simulink model "Lab3"  (Simulink 7.3)
settings: Solver=ode1  SolverMode=SingleTasking  StartTime=0.0  StopTime=5  FixedStep=0.001  RelTol=1e-3
values from neighbouring files (symbols this model uses):
  Beq = 0.0015*6    (= 0.009)    [Sve ikad.m]    (also in matlab.mat = 0.0075)
  den_k = [1 100*a]    [Sve ikad.m]    (also in matlab.mat = [1 286.356023126])
  Eff_G = 0.9    [Sve ikad.m]    (also in matlab.mat)
  Eff_M = 0.69    [Sve ikad.m]    (also in matlab.mat)
  Jeq = 2e-3    (= 0.002)    [Sve ikad.m]    (also in matlab.mat)
  Ke = 0.0076776    [Sve ikad.m]    (also in matlab.mat)
  Kg = 70    [Sve ikad.m]    (also in matlab.mat)
  Km = 0.007683    [Sve ikad.m]    (also in matlab.mat)
  Kp = 41.5    [Sve ikad.m]    (also in matlab.mat = 160)
  num_k = [1*a 100]    [Sve ikad.m]    (also in matlab.mat = [2.86356023126 100])
  Ra = 2.6    [Sve ikad.m]    (also in matlab.mat)
undefined symbols (not defined in the file or in its folder): MultiQ, PCI, Quanser
libraries: rtwinlib x2
settings Model: Creator=Labos  LastModifiedBy=Mehatronicki Sustavi  SimulationMode=external  ExtModeTrigDuration=1000000
settings HardwareCC: ProdIntDivRoundTo=Zero  ProdEndianess=LittleEndian  ProdHWDeviceType=Generic->32-bit x86 compatible
settings RTWCC: SystemTargetFile=rtwin.tlc  TemplateMakefile=rtwin.tmf  Description=Real-Time Windows Target  ProcessScript=rtwin_make_rtw_hook  RTWCompilerOptimization=On
settings CodeAppCC: MaxIdLength=95
settings RTWinTargetCC: TargetFunctionLibrary=ANSI_C  PortableWordSizes=off

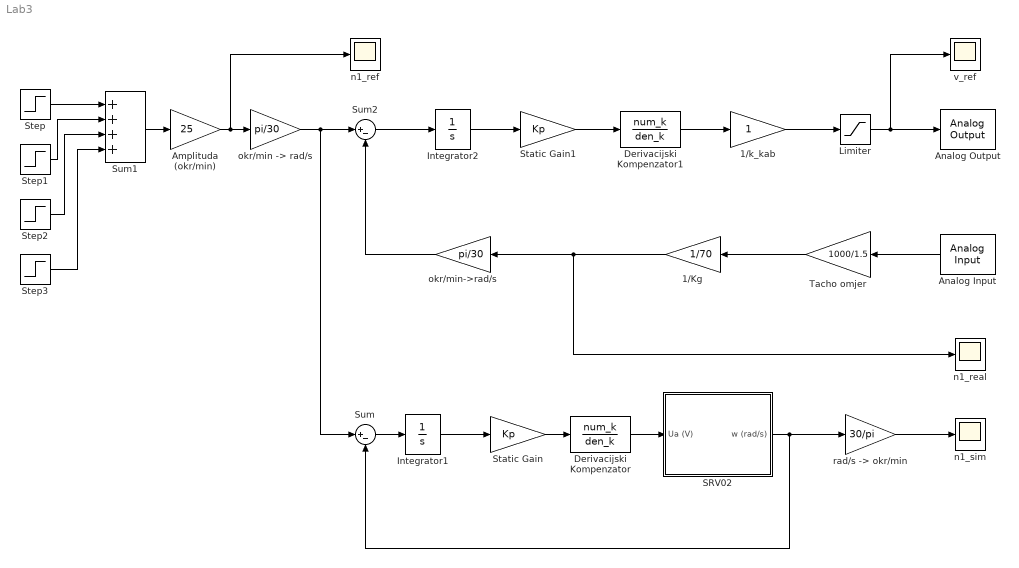
== system Lab3 ==
  1/Kg : Gain  Gain=1/70
  1/k_kab : Gain
  Amplituda (okr/min) : Gain  Gain=25
  Analog Input : rtwinlib/Analog Input  SampleTime=0.001  DrvName=Quanser/MultiQ-PCI  DrvAddress=4294967295  DrvOptions=zeros(1,0)  Channels=4  RangeMode=1  VoltRange=1  DataType=1
      settings: AttributesFormatString=Quanser\nMultiQ-PCI [auto]
  Analog Output : rtwinlib/Analog Output  SampleTime=0.001  DrvName=Quanser/MultiQ-PCI  DrvAddress=4294967295  DrvOptions=zeros(1,0)  Channels=1  RangeMode=1  VoltRange=1  InitialValue=0  FinalValue=0
      settings: AttributesFormatString=Quanser\nMultiQ-PCI [auto]
  Derivacijski Kompenzator : TransferFcn  Numerator=num_k  Denominator=den_k
  Derivacijski Kompenzator1 : TransferFcn  Numerator=num_k  Denominator=den_k
  Integrator1 : Integrator
  Integrator2 : Integrator
  Limiter : Saturate  UpperLimit=6  LowerLimit=-6
  "SRV02 " : Subsystem
  Static Gain : Gain  Gain=Kp
  Static Gain1 : Gain  Gain=Kp
  Step : Step
  Step1 : Step  Time=2  After=-1
  Step2 : Step  Time=3  After=-1
  Step3 : Step  Time=4
  Sum : Sum  Inputs=|+-
  Sum1 : Sum  Inputs=++++
  Sum2 : Sum  Inputs=|+-
  Tacho omjer : Gain  Gain=1000/1.5
  n1_real : Scope
      settings: TimeRange=5  YMin=0  YMax=30  SaveName=n2_real  DataFormat=Array  SampleInput=on
  n1_ref : Scope
      settings: TimeRange=5  YMin=0  YMax=30  SaveName=n2_ref  DataFormat=Array  SampleInput=on
  n1_sim : Scope
      settings: TimeRange=5  YMin=0  YMax=30  SaveName=n2_sim  DataFormat=Array  SampleInput=on
  "okr/min -> rad/s" : Gain  Gain=pi/30
  okr/min->rad/s : Gain  Gain=pi/30
  "rad/s -> okr/min" : Gain  Gain=30/pi
  v_ref : Scope
      settings: TimeRange=5  YMin=0  YMax=30  SaveName=v2_ref  DataFormat=Array  SampleInput=on
  wires:
  "okr/min -> rad/s"/1 -> Sum2/1, Sum/1
  Static Gain/1 -> Derivacijski Kompenzator/1
  Amplituda (okr/min)/1 -> "okr/min -> rad/s"/1, n1_ref/1
  Sum/1 -> Integrator1/1
  Integrator1/1 -> Static Gain/1
  Derivacijski Kompenzator/1 -> "SRV02 "/1(Ua (V))
  "SRV02 "/1(w (rad/s)) -> Sum/2, "rad/s -> okr/min"/1
  "rad/s -> okr/min"/1 -> n1_sim/1
  Sum1/1 -> Amplituda (okr/min)/1
  Step3/1 -> Sum1/4
  Step2/1 -> Sum1/3
  Step1/1 -> Sum1/2
  Step/1 -> Sum1/1
  Static Gain1/1 -> Derivacijski Kompenzator1/1
  Sum2/1 -> Integrator2/1
  Integrator2/1 -> Static Gain1/1
  Derivacijski Kompenzator1/1 -> 1/k_kab/1
  1/k_kab/1 -> Limiter/1
  Limiter/1 -> Analog Output/1, v_ref/1
  okr/min->rad/s/1 -> Sum2/2
  1/Kg/1 -> n1_real/1, okr/min->rad/s/1
  Tacho omjer/1 -> 1/Kg/1
  Analog Input/1 -> Tacho omjer/1

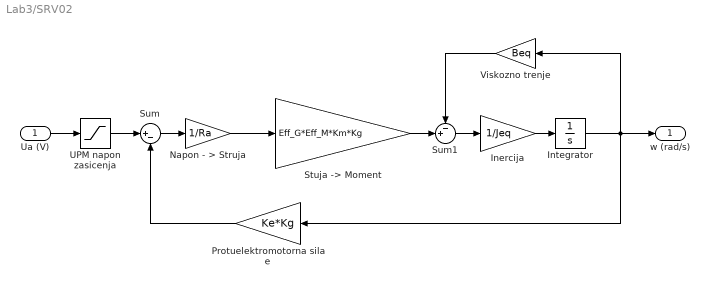
== system Lab3/SRV02  ==
  Ua (V) : Inport
  Inercija : Gain  Gain=1/Jeq
  Integrator : Integrator
  Napon - > Struja : Gain  Gain=1/Ra
  Protuelektromotorna sila e : Gain  Gain=Ke*Kg
  "Stuja -> Moment" : Gain  Gain=Eff_G*Eff_M*Km*Kg
  Sum : Sum  Inputs=|+-
  Sum1 : Sum  Inputs=-+|
  UPM napon zasicenja : Saturate  UpperLimit=6  LowerLimit=-6
  Viskozno trenje : Gain  Gain=Beq
  w (rad/s) : Outport
  wires:
  Sum1/1 -> Inercija/1
  "Stuja -> Moment"/1 -> Sum1/2
  Inercija/1 -> Integrator/1
  UPM napon zasicenja/1 -> Sum/1
  Napon - > Struja/1 -> "Stuja -> Moment"/1
  Ua (V)/1 -> UPM napon zasicenja/1
  Sum/1 -> Napon - > Struja/1
  Viskozno trenje/1 -> Sum1/1
  Protuelektromotorna sila e/1 -> Sum/2
  Integrator/1 -> w (rad/s)/1, Protuelektromotorna sila e/1, Viskozno trenje/1
